simulink model "ORC_test_simu_unregSCIG"  (R2018a)
settings: Solver=FixedStepAuto  StartTime=0.0  StopTime=10  FixedStep=.1  RelTol=1e-4
values from neighbouring files (symbols this model uses):
  A_cond = 50    [Chena_ORC_test_simu_init.m]    (also in ORC_test_simu_init.m = 18.6)
  A_evap = 30    [Chena_ORC_test_simu_init.m]    (also in ORC_test_simu_init.m = 9.3)
  Cx = 620e-05    (= 0.0062)    [Chena_ORC_test_simu_init.m]    (also in ORC_test_simu_init.m = 0.000221048532072; SCIG_Admittance_Balance.m = 6.9e-05; SCIG_Energy_Balance_excitation.m = 1.35135135135; SCIG_Energy_Balance_excitation_sym.m = 5)
  eff_inverter = 0.93    [Chena_ORC_test_simu_init.m]    (also in ORC_test_simu_init.m)
  eff_pump = 0.78    [Chena_ORC_test_simu_init.m]    (also in ORC_Energy_Balance.m = 0.7; ORC_test.m = 0.7; ORC_test_brownfield.m = 0.7; ORC_test_greenfield.m = 0.7)
  eff_turbine = 0.8    [Chena_ORC_test_simu_init.m]    (also in ORC_test_simu_init.m = 0.78)
  f_rated = 60    [Chena_ORC_test_simu_init.m]    (also in ORC_test_simu_init.m; SCIG_Admittance_Balance.m; SCIG_Admittance_test.m; SCIG_Ouazenne.m)
  H_wf_init = 2.6e+05    (= 260000)    [Chena_ORC_test_simu_init.m]    (also in ORC_test_simu_init.m = 230000)
  Lr = 0.252/(2*pi*f_rated)/35    (= 1.9098593171e-05)    [Chena_ORC_test_simu_init.m]    (also in ORC_test_simu_init.m = 0.000132629119243)
  Ls = 0.423/(2*pi*f_rated)/35    (= 3.20583528228e-05)    [Chena_ORC_test_simu_init.m]    (also in ORC_test_simu_init.m = 0.000848826363157)
  m_dot_source = 33.39    [Chena_ORC_test_simu_init.m]    (also in ORC_Energy_Balance.m = 5.7714; ORC_test.m = 12; ORC_test_brownfield.m = 6; ORC_test_greenfield.m = 12)
  m_dot_wf_init = 12    [Chena_ORC_test_simu_init.m]    (also in ORC_test_simu_init.m = 3)
  m_dot_wf_max = 16    [Chena_ORC_test_simu_init.m]
  magCurveV = [98.1532063054068,98.8036071709152,99.4518999785459,100.098037520928,100.741973127402,101.383660677656,102.023054614968,102.660109959042,103.294782318460,103.927027902737,104.556803533993,105.184066658235,105.808775356268,106.430888354220,107.050365033694,107.667165441552,108.281250299330,108.892581012284,109.501119678081,110.106829095126,110.709672770539,111.309614927775,111.906620513896,112.5006 ...(+6146 chars)    [Chena_ORC_test_simu_init.m]    (also in ORC_test_simu_init.m = [21.5410077151772,22.1687511430959,22.7961934111159,23.42344)
  magCurveX = [0.663529769645709,0.663521969965503,0.663500208426959,0.663464444749194,0.663414643227627,0.663350772676200,0.663272806369214,0.663180721982808,0.663074501536138,0.662954131332260,0.662819601898778,0.662670907928276,0.662508048218555,0.662331025612717,0.662139846939116,0.661934522951205,0.661715068267290,0.661481501310239,0.661233844247137,0.660972122928937,0.660696366830103,0.660406608988283,0.6 ...(+6531 chars)    [Chena_ORC_test_simu_init.m]    (also in ORC_test_simu_init.m = [21.5410077151772,21.5637559851946,21.5850104594817,21.60498)
  p_atm = 101325    [Chena_ORC_test_simu_init.m]    (also in ORC_test_simu_init.m)
  pf_grid = 0.9    [Chena_ORC_test_simu_init.m]    (also in ORC_test_simu_init.m)
  poles = 2    [Chena_ORC_test_simu_init.m]    (also in Copy_of_SCIG_Energy_Balance_excitation.m = 4; SCIG_Admittance_Balance.m = 6; SCIG_Admittance_test.m = 6; SCIG_Ouazenne.m)
  Rr = 0.144/35    (= 0.00411428571429)    [Chena_ORC_test_simu_init.m]    (also in ORC_test_simu_init.m = 0.03)
  Rs = 0.148/35    (= 0.00422857142857)    [Chena_ORC_test_simu_init.m]    (also in ORC_test_simu_init.m = 0.018)
  Rx = 0    [Chena_ORC_test_simu_init.m]    (also in Copy_of_SCIG_Energy_Balance_excitation.m = 0.003; ORC_test_simu_init.m; SCIG_Admittance_Balance.m; SCIG_Admittance_test.m)
  Tin_sink = 277.59    [Chena_ORC_test_simu_init.m]    (also in ORC_test_simu_init.m = 278)
  Tin_source = 346.48    [Chena_ORC_test_simu_init.m]    (also in ORC_test_simu_init.m = 368)
  U_cond = 5000    [Chena_ORC_test_simu_init.m]    (also in ORC_test_simu_init.m = 1400)
  U_evap = 4500    [Chena_ORC_test_simu_init.m]    (also in ORC_test_simu_init.m = 1500)
  Vline_rated = 220    [Chena_ORC_test_simu_init.m]    (also in SCIG_Admittance_Balance.m = 6600; SCIG_Admittance_test.m = 6600; SCIG_Ouazenne.m; SCIG_Ouazenne_iterate.m)
  Xx = 1/(2*pi*f_rated*Cx)    (= 0.427835868527)    [Chena_ORC_test_simu_init.m]    (also in Copy_of_SCIG_Energy_Balance_excitation.m = 12; ORC_test_simu_init.m = 12; SCIG_Admittance_Balance.m = Xx(fvIDX); SCIG_Energy_Balance_excitation.m = 1./(Cx.*w_synch))
undefined symbols (not defined in the file or in its folder): handle_sink, handle_source, handle_wf, n_mech_init, n_mech_max, n_mech_min, sigbuilder_block
(part 4 of 4)

== matlab function ORC_test_simu_unregSCIG/Generator/MATLAB Function ==
  data: n_mech input; P_load_out output; P_loss output; Q_loss output; P_load_in input; Vline input; P_mech_needed output; f_e output; Xm output; Vline_out output; f_rated parameter; poles parameter; K_b parameter; K_w parameter; R1 parameter; L1 parameter; R2 parameter; L2 parameter; Cx parameter; magCurveX parameter; magCurveV parameter
function [ P_load_out, P_loss, Q_loss, P_mech_needed, f_e, Xm, Vline_out] = SCIG_Ouazenne_it( n_mech, P_load_in, Vline, f_rated, poles, K_b, K_w, R1, L1, R2, L2, Cx, magCurveX, magCurveV)
%SCIG_ENERGY_BALANCE Summary of this function goes here 
%   This function calcluates the active power (P_loss) losses of a 3-phase 
%   squirrel cage induction generator (SCIG). Also calclulated is the
%   reactive power loss (Q_loss). Induction machines always consume Q
%   (negative Q_out) and the excitation capacitance generates Q (positive
%   Q_out).

%   Circuit diagram of an Asynchronous machine. 
%      Iin>   Ix         I1>        Im        I2>
%              v      R1     jw*X1   v     R2     jw*X2
%     0--------|-----RRRR----XXXX----|----RRRR----XXXX----|
%              |                    E|                    |
%     +        R  Rx               |-|-|                  |
%              R                   |   |                  R
%     Vph      |               Rm  R   X   jw*Xm          R  R2(1-slip)/slip
%              |                   R   X                  R
%     -       CCC  1/jw*Cx         |   |                  R
%              |                   |-|-|                  |
%              |                     |                    |  
%     0--------|---------------------|--------------------|
  
% Inputs:
%   P_load      Three phase active load power in W
%   Q_load      Three phase reactive load power in VAR
%   n_mech      Angular velocity of rotor in rpm
%   f_rated     Rated synchronous frequency in Hz
%   Vline_rated Rated line voltage in V
%   poles       Number of poles
%   K_b         Bearing coefficient 
%   K_w         Windage coefficient
%   R1          Stator resistance in ohm
%   L1          Stator inductance in H
%   R2          Rotor resistance in ohm
%   L2          Rotor inductance in H
%   Rm          Magnetizing resistance of the core in ohm
%   Lm          Magnetizing inductance of the core in L
%   Cx          External Excitation capacitance in F
%
% Outputs:
%   P_loss
%   Q_loss
%   Vph
%   P_mech      Mech power to rotor (P_mech = w_mech*Torque)

var_length = size(n_mech);
P_load_out = zeros(var_length);
% Q_out = zeros(var_length);
P_loss = zeros(var_length);
Q_loss = zeros(var_length);
f_e = zeros(var_length);
Xm = zeros(var_length);
Vline_out = zeros(var_length);


n_synchRated = f_rated*120/poles;
b = n_mech./n_synchRated;

% The mechanical angular velocity
w_mech = 2*pi*n_mech/60;

% calculate reactive impedance from inductance values (X = w*L) and 
% capacitance value (X = 1/(w*C)) at rated frequencies
X1 = 2*pi*f_rated.*L1;
X2 = 2*pi*f_rated.*L2;
Xx = 1./(Cx*2*pi*f_rated);

% calculate friction and windage losses
P_bearing = K_b .* w_mech;
P_windage = K_w .* w_mech.^2;

% calculated the impedance of the load based off power consumed at rated
% line to line voltage
Z_load = LoadImpedance(P_load_in, 0, Vline);
R_load = real(Z_load);

% Calcluate coefficients used to calculated the operating frequency
% relative to the rated frequency. These coefficients can be found in the
% appendix of Analysis of the Isolated Inducution Generator by Ouazenne and
% McPherson.  Note in the text Q2 and Q3 both have a typo which has been
% corrected here.
if R_load < inf
    Rtemp = R1 + R_load;
    
    Q0 = -b*R2*(Rtemp/R_load)^2;
    Q1 = R2*(Rtemp/R_load)^2 + Rtemp*(R2/R_load)^2 + b^2*Rtemp*(X2/R_load)^2;
    Q2 = -2*b*Rtemp*(X2/R_load)^2 - b*R2*((R1/Xx)^2 + (X1/R_load)^2 - 2*(X1/Xx));
    Q3 = R2*((X1/R_load)^2 + (R1/Xx)^2 - 2*(X1/Xx)) + Rtemp*(X2/R_load)^2 + R1*(R2/Xx)^2 + b^2*R1*(X2/Xx)^2;
    Q5 = R2*(X1/Xx)^2 + R1*(X2/Xx)^2;
    Q4 = -b*(Q5 + R1*(X2/Xx)^2);

else
    Q0 = -b*R2;
    Q1 = R2;
    Q2 = - b*R2*((R1/Xx)^2 - 2*(X1/Xx));
    Q3 = R2*((R1/Xx)^2 - 2*(X1/Xx)) + R1*(R2/Xx)^2 + b^2*R1*(X2/Xx);
    Q5 = R2*(X1/Xx)^2 + R1*(X2/Xx)^2;
    Q4 = -b*(Q5 + R1*(X2/Xx)^2);
end

% Calculate all the roots based from the coeffecients
aroots = roots([Q5 Q4 Q3 Q2 Q1 Q0]);

% Ouazzene and McPherson state there should only be one real root
a = real(aroots(end));
% a = aroots(~imag(aroots))
% a = .95;

% Calculate the series equivalent of load and ext. excitation capacitance
RL = R_load*Xx^2/(a*(a^2*R_load^2 + Xx^2));
XL = R_load^2*Xx/(a^2*R_load^2 + Xx^2);

% % calculate the operating frquency
f_e = a*f_rated;

% Calculate impedance of the core base of Ouazenne and McPherson
if R_load < inf
    Xm = ((RL + R1/a)*(X2^2 + (R2/(a-b))^2))/((R2/(a-b))*(X1-XL) - X2*(RL + R1/a));
else
    Xm = ((R1/a)*(X2^2 + (R2/(a-b))^2))/((R2/(a-b))*(X1 - Xx/a^2) - R1*X2/a);
end

% from Xm and magnatization curve calculate internal voltage magnitude
E_f = interp1(magCurveX,magCurveV,Xm,'linear');
% E_f = 240;

% calcluate phase voltage magnitude
if R_load < inf
    Vph = a*E_f/sqrt((1-a^2*(X1/Xx))^2 + a^2*((X1/R_load)^2 + (R1/Xx)^2) + (1 + R1/R_load)^2 - 1);
else
    Vph = a*E_f/sqrt((1-a^2*(X1/Xx))^2 + (a*R1/Xx)^2);
end

Vline_out = Vph*sqrt(3);

% calculate slip from electrical frequency and rotor speed relative to
% rated values
slip = (a-b)/a;


% recalculate reactive impedances for operating frequency
X1 = 2*pi*f_e.*L1;
X2 = 2*pi*f_e.*L2;
Xx = 1./(Cx*2*pi*f_e);
Xm = Xm*f_e/f_rated;

% calculate stator, rotor, core, and excitation per-unit impedances
Z_stator = R1 + 1i*X1;   % R1 and X1 in series
% Z_core = 1./(1./Rm + 1./(1i*Xm));   % Rm and Xm in parallel
Z_core = 1i*Xm;
Z_rotor = R2./slip + 1i*X2;   % R2/slip and X2 in series
Z_machine = Z_stator + 1./(1./Z_core + 1./Z_rotor);
Z_excite = Xx/(1i);   

% Calculate stator current 
I1 = Vph/Z_machine;

% Calculate excitation current
Ix = Vph./Z_excite;

% Calculate internal voltage
E = Vph - I1*Z_stator;

% Calculate magnetizing current
Im = E./Z_core;

% Calculate rotor current
I2 = E./Z_rotor;

% Calculate load current
Iload = Vph./Z_load;

 
% Calculate active and reactive power losses in the asynch machine
Q_loss_rotor = 3*abs(I2).^2.*X2;
P_RCL = 3*abs(I2).^2.*R2;

Q_loss_stator = 3*abs(I1).^2.*X1;
P_SCL = 3*abs(I1).^2.*R1;

Q_loss_core = 3*abs(E).^2./(Xm);
P_core =0;% 3*abs(E).^2./Rm;

if any(Ix)
%     Sometimes when there is an infinite impedance matlab will calculate
%     NaN even though there is 0 current. This if/else ensures the power
%     calculations result in 0 when current is 0.
    Q_loss_excitation = -3*abs(Ix).^2.*(Xx);
else
    Q_loss_excitation = 0;
end

 
% Calculate total real and reactive powers. Reactive power is only
% consumed not generated therefore Q_out should be negative.
Q_loss(:) = (Q_loss_core + Q_loss_rotor + Q_loss_stator);% + Q_loss.excitation;
% P_out = P_conv -(P_excitation + P_RCL + P_SCL + P_core);

% Output real losses in stucture
P_loss_mech = P_bearing + P_windage;
P_loss_copper = P_RCL + P_SCL;
P_loss_core = P_core;
P_loss(:) = P_bearing + P_windage + P_RCL + P_SCL + P_core;

P_load_out(:) = real(3*abs(Vph)^2/conj(Z_load));
P_conv = -3.*abs(I2).^2.*R2.*(1-slip)./slip;
P_mech_needed = P_conv + P_bearing + P_windage;
% Q_out(:) = zeros(var_length);%Q_loss + Q_loss_excitation;
end
%
